simulink model "Comparaison_Simscape_FonctionTransfert"  (R2015a)
settings: Solver=ode23t  StartTime=0.0  StopTime=10  FixedStep=0.00025  RelTol=1e-3
InitFcn:
  | load('LeftOutput_Measures.mat');
  | load('LeftOutput_Measures.mat');
  | Parametres_Rover
undefined symbols (not defined in the file): KL, TdL, TL
libraries: SingleMotor_V_to_rads x1, SingleMotor_Duty_to_inc x1
settings Model: Creator=tbaroche  LastModifiedBy=tbaroche

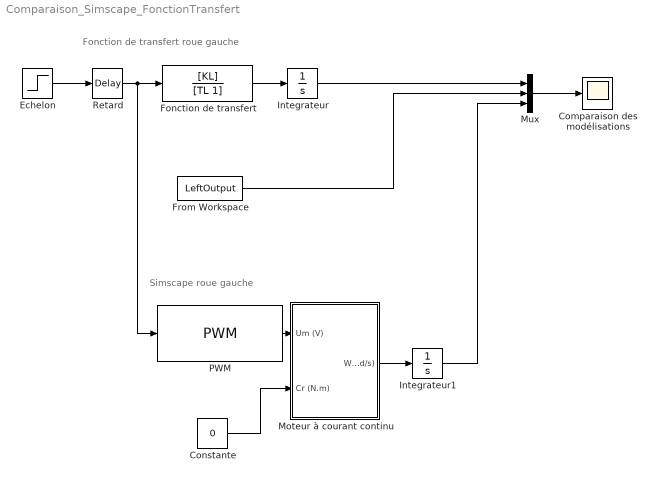
== system Comparaison_Simscape_FonctionTransfert ==
  note: Simscape roue gauche
  note: Fonction de transfert roue gauche
  Comparaison des modélisations : Scope
      settings: TimeRange=10  YMin=1500  YMax=9000
  Constante : Constant  Value=0
  Echelon : Step  Time=3  After=50  SampleTime=0
  Fonction de transfert : TransferFcn  Numerator=[KL]  Denominator=[TL 1]
  From Workspace : FromWorkspace  VariableName=LeftOutput  SampleTime=0
  Integrateur : Integrator
  Integrateur1 : Integrator
  Moteur à courant continu : Subsystem  BlockChoice=Modèle Simscape
      link override Modèle Simscape/Simulink-PS Converter/input0: OutDataTypeStr=double  PortDimensions=-1
      link override Modèle Simscape/Simulink-PS Converter1/input0: OutDataTypeStr=double  PortDimensions=-1
      link override "SimElectronics Model ": Kphi_lib=Kphi  Rm_lib=Rm  Lm_lib=Lm  bm_lib=bm  Jm_lib=Jm
      link override Simscape Model/Simulink-PS Converter/input0: OutDataTypeStr=double  PortDimensions=-1
      link override Simscape Model/Simulink-PS Converter1/input0: OutDataTypeStr=double  PortDimensions=-1
      settings: AttributesFormatString=%<BlockChoice>  TemplateBlock=SingleMotor_V_to_rads/DC Motor  MemberBlocks=Modèle Simscape,Modèle Simulink
  Mux : Mux  Inputs=3
  PWM : SingleMotor_Duty_to_inc/PWM  FreqTriangle=FreqPWM
  Retard : TransportDelay  DelayTime=TdL
  wires:
  Mux/1 -> Comparaison des modélisations/1
  Integrateur/1 -> Mux/1
  From Workspace/1 -> Mux/2
  Fonction de transfert/1 -> Integrateur/1
  Echelon/1 -> Retard/1
  Integrateur1/1 -> Mux/3
  Constante/1 -> Moteur à courant continu/2(Cr (N.m))
  PWM/1 -> Moteur à courant continu/1(Um (V))
  Moteur à courant continu/1(Wm (rad/s)) -> Integrateur1/1
  Retard/1 -> PWM/1, Fonction de transfert/1

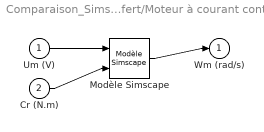
== system Comparaison_Simscape_FonctionTransfert/Moteur à courant continu ==
  Um (V) : Inport
  Cr (N.m) : Inport  Port=2
  Modèle Simscape : SingleMotor_V_to_rads/Modèle Simscape  Kphi_lib=Kphi  Rm_lib=Rm  Lm_lib=Lm  bm_lib=bm  Jm_lib=Jm
  Wm (rad/s) : Outport
  wires:
  Um (V)/1 -> Modèle Simscape/1
  Cr (N.m)/1 -> Modèle Simscape/2
  Modèle Simscape/1 -> Wm (rad/s)/1
